simulink model "postSNR_ver"  (R2019a)
settings: Solver=VariableStepAuto  StartTime=0.0  StopTime=(nSamp - 1)*Ts  RelTol=1e-3
InitFcn:
  | postSNR_verScript;
StopFcn:
  | % Simulation Stuff
  | postOut  = out.postSNR.signals.values(:, 1:FFT_size);
  | 
  | figure(2);
  | stem(1:FFT_size, postOut(1,:), '*');
  | hold on;
  | stem(1:FFT_size, postSNRa(1,:), 'o');
  | hold off;
  | xlabel('Samples');
  | legend('Sim Data', 'Script Data');
  | title('PostSNR Outputs: Simulation vs Script');
  | print('postSNR_Output', '-djpeg');
values from neighbouring files (symbols this model uses):
  FFT_size = 64    [FIR_filterTestm.m]    (also in JMAP_INIT.m; blockVerification.m; block_verScript.m; ksi_verScript.m)
  Ts = 1/Fs    (= 2.08333333333e-05)    [FIR_filterTestm.m]    (also in JMAP_INIT.m; blockVerification.m; block_verScript.m; ksi_verScript.m)
libraries: simulink x1
settings Model: Creator=Showi  LastModifiedBy=Showi

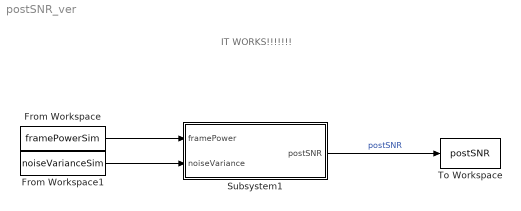
== system postSNR_ver ==
  note: IT WORKS!!!!!!!
  From Workspace : FromWorkspace  VariableName=framePowerSim  SampleTime=Ts  Interpolate=off  OutputAfterFinalValue=Setting to zero
  From Workspace1 : FromWorkspace  VariableName=noiseVarianceSim  SampleTime=Ts  Interpolate=off  OutputAfterFinalValue=Setting to zero
  Subsystem1 : Subsystem
  To Workspace : ToWorkspace  VariableName=postSNR  SaveFormat=Structure With Time  SampleTime=-1
  wires:
  Subsystem1/1(postSNR) -> To Workspace/1  "postSNR"
  From Workspace/1 -> Subsystem1/1(framePower)
  From Workspace1/1 -> Subsystem1/2(noiseVariance)

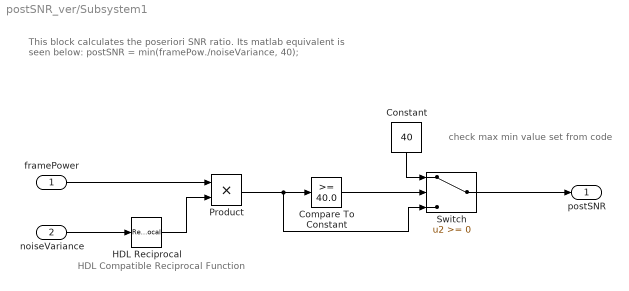
== system postSNR_ver/Subsystem1 ==
  note: This block calculates the poseriori SNR ratio.
      |
      | Its matlab equivalent is seen below:
      | 	postSNR = min(framePow./noiseVariance, 40);
  note: HDL Compatible Reciprocal Function
  note: check max min value set from code
  framePower : Inport
  noiseVariance : Inport  Port=2
  Compare To Constant : simulink/Logic and Bit Operations/Compare To Constant  relop=>=  const=40.0  OutDataTypeStr=boolean
  Constant : Constant  Value=40  SampleTime=-1
  HDL Reciprocal : Reciprocal
  Product : Product  Inputs=**
  Switch : Switch
  postSNR : Outport
  wires:
  noiseVariance/1 -> HDL Reciprocal/1
  framePower/1 -> Product/1
  Product/1 -> Switch/3, Compare To Constant/1
  Switch/1 -> postSNR/1
  HDL Reciprocal/1 -> Product/2
  Compare To Constant/1 -> Switch/2
  Constant/1 -> Switch/1
